simulink model "Autopilot_q_full_5may_new1"  (R2020a)
settings: Solver=ode4  StartTime=0.0  StopTime=300  FixedStep=0.01  RelTol=1e-3
undefined symbols (not defined in the file or in its folder): Aero_cofficients, Atmosphere_pert, Atmospheric_model, Counter_sensor_model, Earth, error_global, flags_global, Guidance_Flags_global, INT_global, param_guidance, Payload_data, Plane_state_mode_finish_catcher_ftr_mode, Plane_state_mode_finish_catcher_fw_mode, Plane_state_mode_finish_catcher_q_mode, Plane_state_mode_finish_catcher_rtr_mode, Plane_state_store, propulsion_model, propulsion_model_int, Structural_data, Thrust_data_store, time_global, WGS84, Wind_data, Wind_model_int, Wind_pert_factor
libraries: simulink x33, aerolibactuator x15, cstblocks x3, aerolibatmos2 x2, aerolibfltsims x1, aerolibtransform2 x1, shared6dof x1
(part 1 of 10)
settings Model: SimulationMode=accelerator  Creator=rrpat  LastModifiedBy=VTOL_HYD
settings DataIOCC: ReturnWorkspaceOutputs=off
settings DebuggingCC: ArithmeticOperatorsInVariantConditions=warning
settings SFSimCC: CustomCodeUndefinedFunction=UseInterfaceOnly

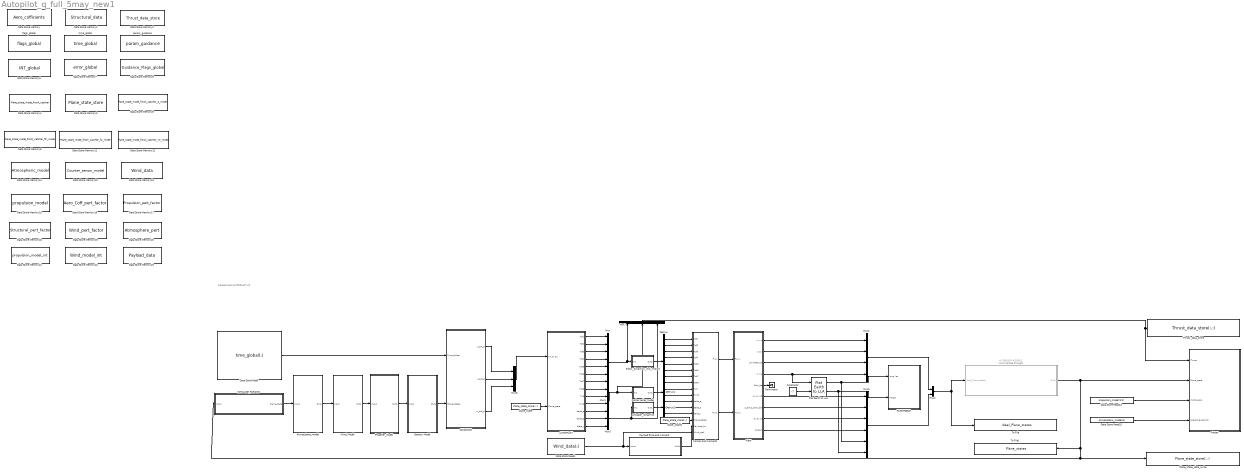
== system Autopilot_q_full_5may_new1 ==
  note: AKSHAYAAN AUTOPILOT V2
  "AUTOPILOT " : Subsystem
  Actuator_dynamics : Subsystem
  All SENSOR MODEL2 : Subsystem  Commented=through  TreatAsAtomicUnit=on
  Atmosphere_model : Subsystem
  Battery Model : Subsystem
  Constant2 : Constant  Value=-7
  Data Store Memory : DataStoreMemory  Priority=1  DataStoreName=Aero_cofficients  ReadBeforeWriteMsg=warning  WriteAfterWriteMsg=warning  WriteAfterReadMsg=warning  InitialValue=[0 0 0 0 0 0 0 0 0;0 0 0 0 0 0 0 0 0;0 0 0 0 0 0 0 0 0;0 0 0 0 0 0 0 0 0;0 0 0 0 0 0 0 0 0;0 0 0 0 0 0 0 0 0]  VectorParams1D=off  ShowAdditionalParam=off
  Data Store Memory1 : DataStoreMemory  Priority=2  DataStoreName=Structural_data  ReadBeforeWriteMsg=warning  WriteAfterWriteMsg=warning  WriteAfterReadMsg=warning  InitialValue=[25.0,0,0,0,0,0,0,0,0,0,0,0,0,0,0,0,0,0,0,0,0,0,0,0]  VectorParams1D=off  ShowAdditionalParam=off  OutDataTypeStr=double
  Data Store Memory10 : DataStoreMemory  Priority=17  DataStoreName=Counter_sensor_model  ReadBeforeWriteMsg=warning  WriteAfterWriteMsg=warning  WriteAfterReadMsg=warning  InitialValue=[0,0,0,0,1,1,1,1]  ShowAdditionalParam=off
  Data Store Memory11 : DataStoreMemory  Priority=15  DataStoreName=Plane_state_mode_finish_catcher_fw_mode  ReadBeforeWriteMsg=warning  WriteAfterWriteMsg=warning  WriteAfterReadMsg=warning  InitialValue=[0,0,0,0,0,0,0,0,0,0,0,0,0,0]  ShowAdditionalParam=off
  Data Store Memory12 : DataStoreMemory  Priority=14  DataStoreName=Plane_state_mode_finish_catcher_rtr_mode  ReadBeforeWriteMsg=warning  WriteAfterWriteMsg=warning  WriteAfterReadMsg=warning  InitialValue=[0,0,0,0,0,0,0,0,0,0,0,0,0,0]  ShowAdditionalParam=off
  Data Store Memory13 : DataStoreMemory  Priority=18  DataStoreName=Wind_data  ReadBeforeWriteMsg=warning  WriteAfterWriteMsg=warning  WriteAfterReadMsg=warning  InitialValue=[0,0,0]  ShowAdditionalParam=off
  Data Store Memory14 : DataStoreMemory  Priority=16  DataStoreName=Atmospheric_model  ReadBeforeWriteMsg=warning  WriteAfterWriteMsg=warning  WriteAfterReadMsg=warning  InitialValue=[0,0,0,0]  ShowAdditionalParam=off
  Data Store Memory15 : DataStoreMemory  Priority=19  DataStoreName=propulsion_model  ReadBeforeWriteMsg=warning  WriteAfterWriteMsg=warning  WriteAfterReadMsg=warning  InitialValue=[0,0,0,0]  ShowAdditionalParam=off
  Data Store Memory16 : DataStoreMemory  Priority=20  DataStoreName=Aero_Coff_pert_factor  ReadBeforeWriteMsg=warning  WriteAfterWriteMsg=warning  WriteAfterReadMsg=warning  InitialValue=[1 1 1 1 1 1 1 1 1;1 1 1 1 1 1 1 1 1;1 1 1 1 1 1 1 1 1;1 1 1 1 1 1 1 1 1;1 1 1 1 1 1 1 1 1;1 1 1 1 1 1 1 1 1]  VectorParams1D=off  ShowAdditionalParam=off
  Data Store Memory17 : DataStoreMemory  Priority=21  DataStoreName=Propulsion_pert_factor  ReadBeforeWriteMsg=warning  WriteAfterWriteMsg=warning  WriteAfterReadMsg=warning  InitialValue=[1,1,1,1]  ShowAdditionalParam=off
  Data Store Memory18 : DataStoreMemory  Priority=22  DataStoreName=Structural_pert_factor  ReadBeforeWriteMsg=warning  WriteAfterWriteMsg=warning  WriteAfterReadMsg=warning  InitialValue=[1,1,1,1,1,1,1,1,1,1,1,1,1,1,1,1,1,1,1,1,1,1,1,1]  VectorParams1D=off  ShowAdditionalParam=off  OutDataTypeStr=double
  Data Store Memory19 : DataStoreMemory  Priority=23  DataStoreName=Wind_pert_factor  ReadBeforeWriteMsg=warning  WriteAfterWriteMsg=warning  WriteAfterReadMsg=warning  InitialValue=[1,1,1]  ShowAdditionalParam=off
  Data Store Memory2 : DataStoreMemory  Priority=3  DataStoreName=Thrust_data_store  ReadBeforeWriteMsg=warning  WriteAfterWriteMsg=warning  WriteAfterReadMsg=warning  InitialValue=[0,0,0,0,0,0,0,0,0,0,0,0,0]  VectorParams1D=off  ShowAdditionalParam=off
  Data Store Memory20 : DataStoreMemory  Priority=24  DataStoreName=Atmosphere_pert  ReadBeforeWriteMsg=warning  WriteAfterWriteMsg=warning  WriteAfterReadMsg=warning  InitialValue=[1,1,1,1]  ShowAdditionalParam=off
  Data Store Memory21 : DataStoreMemory  Priority=27  DataStoreName=propulsion_model_int  ReadBeforeWriteMsg=warning  WriteAfterWriteMsg=warning  WriteAfterReadMsg=warning  InitialValue=[0,0,0,0]  ShowAdditionalParam=off
  Data Store Memory22 : DataStoreMemory  Priority=26  DataStoreName=Wind_model_int  ReadBeforeWriteMsg=warning  WriteAfterWriteMsg=warning  WriteAfterReadMsg=warning  InitialValue=[0,0,0,0,0,0,0,0,0,0]  ShowAdditionalParam=off
  Data Store Memory23 : DataStoreMemory  Priority=25  DataStoreName=Payload_data  ReadBeforeWriteMsg=warning  WriteAfterWriteMsg=warning  WriteAfterReadMsg=warning  InitialValue=[0,0,0,0,0,0,0,0,0,0,0,0,0,0,0,0,0,0,0,0,0,0,0,0,0,0,0,0,0,0]  ShowAdditionalParam=off
  Data Store Memory3 : DataStoreMemory  Priority=11  DataStoreName=Plane_state_store  ReadBeforeWriteMsg=warning  WriteAfterWriteMsg=warning  WriteAfterReadMsg=warning  InitialValue=[0,0,0,0,0,0,0,0,0,0,0,0,0,0,0,0,0,0,0,0,0,0,0,0,0,0,0]  VectorParams1D=off  ShowAdditionalParam=off
  Data Store Memory4 : DataStoreMemory  Priority=10  DataStoreName=Plane_state_mode_finish_catcher  ReadBeforeWriteMsg=warning  WriteAfterWriteMsg=warning  WriteAfterReadMsg=warning  InitialValue=[0,0,0,0,0,0,0,0,0,0,0,0,0,0]  ShowAdditionalParam=off
  Data Store Memory5 : DataStoreMemory  Priority=7  DataStoreName=INT_global  ReadBeforeWriteMsg=warning  WriteAfterWriteMsg=warning  WriteAfterReadMsg=warning  InitialValue=[0,0,0,0,0,0,0,0,0,0,0,0,0,0]  ShowAdditionalParam=off
  Data Store Memory6 : DataStoreMemory  Priority=9  DataStoreName=Guidance_Flags_global  ReadBeforeWriteMsg=warning  WriteAfterWriteMsg=warning  WriteAfterReadMsg=warning  InitialValue=[0,0,0,0,0,0,0,0,0,0,0,0,0,0,0,0,0,0,0,0,0,0,0,0,0,0,0,0,0,0,0,0,0,0,0,0,0,0,0,0,0,0,0,0,0,0,0,0,0,0,0]  VectorParams1D=off  ShowAdditionalParam=off
  Data Store Memory7 : DataStoreMemory  Priority=8  DataStoreName=error_global  ReadBeforeWriteMsg=warning  WriteAfterWriteMsg=warning  WriteAfterReadMsg=warning  InitialValue=[0,0,0,0,0,0]  ShowAdditionalParam=off
  Data Store Memory8 : DataStoreMemory  Priority=12  DataStoreName=Plane_state_mode_finish_catcher_q_mode  ReadBeforeWriteMsg=warning  WriteAfterWriteMsg=warning  WriteAfterReadMsg=warning  InitialValue=[0,0,0,0,0,0,0,0,0,0,0,0,0,0]  ShowAdditionalParam=off
  Data Store Memory9 : DataStoreMemory  Priority=13  DataStoreName=Plane_state_mode_finish_catcher_ftr_mode  ReadBeforeWriteMsg=warning  WriteAfterWriteMsg=warning  WriteAfterReadMsg=warning  InitialValue=[0,0,0,0,0,0,0,0,0,0,0,0,0,0]  ShowAdditionalParam=off
  Data Store Read : DataStoreRead  DataStoreName=time_global  DataStoreElements=time_global(:)
  Data Store Read1 : DataStoreRead  DataStoreName=Wind_data  SampleTime=0.01  DataStoreElements=Wind_data(:)
  Data Store Read13 : DataStoreRead  DataStoreName=propulsion_model  DataStoreElements=propulsion_model(1:2)
  Data Store Read15 : DataStoreRead  DataStoreName=Atmospheric_model  DataStoreElements=Atmospheric_model(4)
  Demux : Demux  Outputs=8
  Demux1 : Demux  Outputs=2
  Demux2 : Demux  Outputs=3
  FLIGHTGEAR : Subsystem
  Flat Earth to LLA : aerolibtransform2/Flat Earth to LLA  units=Metric (MKS)  ptype=Earth (WGS84)  F=1/298.257223563  R=6378137  refPosPort=off  LL0=[37.6188056,-122.3754167 ]  psi=0
  Forces and moments : Subsystem
  GUIDANCE : Subsystem
  INITIALISE_PARAMS : Subsystem  Priority=28
  Mux : Mux  Inputs=8
  Mux1 : Mux  Inputs=2
  Mux2 : Mux
  Mux3 : Mux  Inputs=6
  Mux4 : Mux  Inputs=2
  Mux5 : Mux  Inputs=3
  Mux6 : Mux  Inputs=3
  Mux7 : Mux  Inputs=3
  Payload force and moment : Subsystem
  Plane_state_data_write : DataStoreWrite  DataStoreName=Plane_state_store  DataStoreElements=Plane_state_store(:,:)
  Plant : Subsystem
  Plotter : Subsystem
  Propeller_Model : Subsystem
  Pusher.puller model : Subsystem
  Rotor_dynamics_vtol_motors : Subsystem
  Terminator : Terminator
  Thrust_data_store : DataStoreWrite  DataStoreName=Thrust_data_store  DataStoreElements=Thrust_data_store(:,:)
  To File : ToFile  Filename=ideal_Plane_states
  To File1 : ToFile  Filename=Plane_states  SaveFormat=Timeseries
  Wind_Model : Subsystem
  flags_global : DataStoreMemory  Priority=4  DataStoreName=flags_global  ReadBeforeWriteMsg=warning  WriteAfterWriteMsg=warning  WriteAfterReadMsg=warning  InitialValue=[0,0,0,0,0,0,0,0,0,0,0,0,0,0,0,1,1,1,1,1,1,0,0,0,1,1,0,0]  ShowAdditionalParam=off
  param_guidance : DataStoreMemory  Priority=6  DataStoreName=param_guidance  ReadBeforeWriteMsg=warning  WriteAfterWriteMsg=warning  WriteAfterReadMsg=warning  InitialValue=[0,0,0,0]  ShowAdditionalParam=off
  plane_state : DataStoreRead  DataStoreName=Plane_state_store  SampleTime=0.01  DataStoreElements=Plane_state_store(:,:)
  plane_state1 : DataStoreRead  DataStoreName=Plane_state_store  SampleTime=0.01  DataStoreElements=Plane_state_store(:,:)
  time_global : DataStoreMemory  Priority=5  DataStoreName=time_global  ReadBeforeWriteMsg=warning  WriteAfterWriteMsg=warning  WriteAfterReadMsg=warning  InitialValue=[0,0,0,0,0,0,0,0,0]  ShowAdditionalParam=off
  wires:
  "AUTOPILOT "/6(Tzb6) -> Mux/6
  Demux/3 -> Forces and moments/3("Tzf3 ")
  Plant/9(Output) -> Mux3/4
  INITIALISE_PARAMS/1(Plane_state) -> Atmosphere_model/1(Input)
  "AUTOPILOT "/5(Tzb5) -> Mux/5
  Demux2/3 -> Forces and moments/13(delta_r)
  Data Store Read15/1 -> Plotter/4(operating_density)
  Demux/7 -> Forces and moments/7(Tzb7)
  Data Store Read13/1 -> Plotter/3(motor_para)
  Pusher.puller model/1(Out1) -> Demux1/1
  Plant/8(ax,ay,az) -> Mux3/3
  Flat Earth to LLA/1 -> FLIGHTGEAR/1("long, lat"), Mux3/5
  Demux1/1 -> Forces and moments/9(Tx9)
  Demux/8 -> Forces and moments/8(Tzb8)
  Demux/4 -> Forces and moments/4(Tzf4)
  Mux7/1 -> Thrust_data_store/1, Plotter/1(Thrust)
  Demux/1 -> Forces and moments/1(Tzf1)
  Mux6/1 -> "AUTOPILOT "/1(ax,ay,az)
  Mux5/1 -> Mux7/3, Actuator_dynamics/1(In1)
  Demux1/2 -> Forces and moments/10(Tx10)
  Mux/1 -> Mux7/1, Rotor_dynamics_vtol_motors/1(In1)
  Forces and moments/1(Fxyz) -> Plant/1(Fxyz)
  Demux/5 -> Forces and moments/5(Tzb5)
  Demux/6 -> Forces and moments/6(Tzb6)
  "AUTOPILOT "/7(Tzb7) -> Mux/7
  Forces and moments/2(Mxyz) -> Plant/2(Mxyz)
  GUIDANCE/1(u_dot_d) -> Mux6/1
  "AUTOPILOT "/11(delta_e) -> Mux5/1
  GUIDANCE/3(w_dot_d) -> Mux6/3
  "AUTOPILOT "/8(Tzb8) -> Mux/8
  Mux3/1 -> Mux4/2
  Actuator_dynamics/1(Out1) -> Demux2/1
  "AUTOPILOT "/13(delta_r) -> Mux5/3
  "AUTOPILOT "/10(Tx10) -> Mux1/2
  "AUTOPILOT "/12(delta_a) -> Mux5/2
  Rotor_dynamics_vtol_motors/1(Out1) -> Demux/1
  Demux2/1 -> Forces and moments/11(delta_e)
  "AUTOPILOT "/4(Tzf4) -> Mux/4
  Mux1/1 -> Pusher.puller model/1(In1), Mux7/2
  Plant/5(Dcm_be) -> Terminator/1
  Plant/3(phi,theta,psi) -> Mux2/3
  Demux2/2 -> Forces and moments/12(delta_a)
  Plant/1(u,v,w) -> Mux2/1
  "AUTOPILOT "/2(Tzf2) -> Mux/2
  Plant/2(p,q,r) -> Mux2/2
  "AUTOPILOT "/1(Tzf1) -> Mux/1
  "AUTOPILOT "/9(Tx9) -> Mux1/1
  Flat Earth to LLA/2 -> Mux3/6, FLIGHTGEAR/2(height)
  Plant/4(X,Y,Z) -> Mux2/4, Flat Earth to LLA/1
  Plant/7(p_dot,q_dot,r_dot) -> Mux3/2
  Demux/2 -> Forces and moments/2(Tzf2)
  Data Store Read/1 -> GUIDANCE/1(Time global)
  Constant2/1 -> Flat Earth to LLA/2
  GUIDANCE/2(v_dot_d) -> Mux6/2
  Plant/6(VX,VY,VZ) -> Mux3/1
  "AUTOPILOT "/3(Tzf3) -> Mux/3
  Mux2/1 -> Mux4/1
  Mux4/1 -> All SENSOR MODEL2/1(ideal_Plane_states), To File/1
  Data Store Read1/1 -> Forces and moments/16(Wind_ned), Payload force and moment/1(Input)
  Payload force and moment/1(Out1) -> Forces and moments/15(Payload_fm)
  All SENSOR MODEL2/1(Out1) -> Plane_state_data_write/1, INITIALISE_PARAMS/1(Input), To File1/1, Plotter/2(Plane_state)
  Atmosphere_model/1(Out1) -> Wind_Model/1(Input)
  Propeller_Model/1(Out1) -> Battery Model/1(Input)
  Wind_Model/1(Out1) -> Propeller_Model/1(Input)
  Battery Model/1(Out1) -> GUIDANCE/2(Plane_states)
  plane_state/1 -> "AUTOPILOT "/2(Plane_state)
  plane_state1/1 -> Forces and moments/14(Plane_states)

== system Autopilot_q_full_5may_new1/AUTOPILOT  ==
  ax,ay,az : Inport  SampleTime=0.01
  Plane_state : Inport  Port=2  SampleTime=0.01
  Autopilot Fixed wing mode : Subsystem  TreatAsAtomicUnit=on
  Autopilot Quad mode : Subsystem  TreatAsAtomicUnit=on
  Autopilot Transition mode : Subsystem  TreatAsAtomicUnit=on
  Data Store Read : DataStoreRead  DataStoreName=flags_global  SampleTime=0.01  DataStoreElements=flags_global(3)
  Data Store Read1 : DataStoreRead  DataStoreName=flags_global  SampleTime=0.01  DataStoreElements=flags_global(4)
  Data Store Read2 : DataStoreRead  DataStoreName=flags_global  SampleTime=0.01  DataStoreElements=flags_global(5)
  Demux : Demux  Outputs=13
  Display : Display
  Display1 : Display
  Display2 : Display
  If : If  NumInputs=3  IfExpression=u1 == 1  ElseIfExpressions=u2 == 1, u3==1  ShowElse=off
  Mux : Mux  Inputs=13
  Mux1 : Mux  Inputs=13
  Mux2 : Mux  Inputs=13
  Subsystem : Subsystem
  Switch : Switch  Criteria=u2 ~= 0
  Switch1 : Switch  Criteria=u2 ~= 0
  Tzf1 : Outport  VectorParamsAs1DForOutWhenUnconnected=off
  Tzf2 : Outport  Port=2  VectorParamsAs1DForOutWhenUnconnected=off
  Tzf3 : Outport  Port=3  VectorParamsAs1DForOutWhenUnconnected=off
  Tzf4 : Outport  Port=4  VectorParamsAs1DForOutWhenUnconnected=off
  Tzb5 : Outport  Port=5  VectorParamsAs1DForOutWhenUnconnected=off
  Tzb6 : Outport  Port=6  VectorParamsAs1DForOutWhenUnconnected=off
  Tzb7 : Outport  Port=7  VectorParamsAs1DForOutWhenUnconnected=off
  Tzb8 : Outport  Port=8  VectorParamsAs1DForOutWhenUnconnected=off
  Tx9 : Outport  Port=9  VectorParamsAs1DForOutWhenUnconnected=off
  Tx10 : Outport  Port=10  VectorParamsAs1DForOutWhenUnconnected=off
  delta_e : Outport  Port=11  VectorParamsAs1DForOutWhenUnconnected=off
  delta_a : Outport  Port=12  VectorParamsAs1DForOutWhenUnconnected=off
  delta_r : Outport  Port=13  VectorParamsAs1DForOutWhenUnconnected=off
  wires:
  Plane_state/1 -> Autopilot Fixed wing mode/2(Plane_states), Autopilot Transition mode/2(Plane_state), Autopilot Quad mode/2(Plane_states)
  ax,ay,az/1 -> Autopilot Fixed wing mode/1(ax_d,ay_d,az_d), Autopilot Quad mode/1(ax_d,ay_d,az_d), Autopilot Transition mode/1(ax,ay,az)
  If/1 -> Autopilot Quad mode/Action
  If/3 -> Autopilot Fixed wing mode/Action
  Autopilot Quad mode/1(Tzf1) -> Mux/1
  Autopilot Quad mode/2(Tzf2) -> Mux/2
  Autopilot Quad mode/3(Tzf3) -> Mux/3
  Autopilot Quad mode/4(Tzf4) -> Mux/4
  Autopilot Quad mode/5(Tzb5) -> Mux/5
  Autopilot Quad mode/6(Tzb6) -> Mux/6
  Autopilot Quad mode/7(Tzb7) -> Mux/7
  Autopilot Quad mode/8(Tzb8) -> Mux/8
  Autopilot Quad mode/9(Tx9) -> Mux/9
  Autopilot Quad mode/10(Tx10) -> Mux/10
  Autopilot Quad mode/11(delta_e) -> Mux/11
  Autopilot Quad mode/12(delta_a) -> Mux/12
  Autopilot Quad mode/13(delta_r) -> Mux/13
  Autopilot Transition mode/1(Tzf1) -> Mux1/1
  Autopilot Transition mode/2(Tzf2) -> Mux1/2
  Autopilot Transition mode/3(Tzf3) -> Mux1/3
  Autopilot Transition mode/4(Tzf4) -> Mux1/4
  Autopilot Transition mode/5(Tzb5) -> Mux1/5
  Autopilot Transition mode/6(Tzb6) -> Mux1/6
  Autopilot Transition mode/7(Tzb7) -> Mux1/7
  Autopilot Transition mode/8(Tzb8) -> Mux1/8
  Autopilot Transition mode/9(Tx9) -> Mux1/9
  Autopilot Transition mode/10(Tx10) -> Mux1/10
  Autopilot Transition mode/11(delta_e) -> Mux1/11
  Autopilot Transition mode/12(delta_a) -> Mux1/12
  Autopilot Transition mode/13(delta_r) -> Mux1/13
  Mux/1 -> Switch/1
  Subsystem/1(Out1) -> Display1/1, If/1, Switch/2
  Subsystem/2(Out2) -> If/2, Display2/1
  Switch1/1 -> Switch/3
  Switch/1 -> Demux/1
  Demux/8 -> Tzb8/1
  Demux/2 -> Tzf2/1
  Demux/10 -> Tx10/1
  Demux/6 -> Tzb6/1
  Demux/5 -> Tzb5/1
  Demux/7 -> Tzb7/1
  Demux/4 -> Tzf4/1
  Demux/11 -> delta_e/1
  Demux/3 -> Tzf3/1
  Demux/9 -> Tx9/1
  Demux/1 -> Tzf1/1
  Demux/13 -> delta_r/1
  Demux/12 -> delta_a/1
  Subsystem/3(Out3) -> Display/1, Switch1/2, If/3
  If/2 -> Autopilot Transition mode/Action
  Autopilot Fixed wing mode/1(Tzf1) -> Mux2/1
  Autopilot Fixed wing mode/2(Tzf2) -> Mux2/2
  Autopilot Fixed wing mode/3(Tzf3) -> Mux2/3
  Autopilot Fixed wing mode/4(Tzf4) -> Mux2/4
  Autopilot Fixed wing mode/5(Tzb5) -> Mux2/5
  Autopilot Fixed wing mode/6(Tzb6) -> Mux2/6
  Autopilot Fixed wing mode/7(Tzb7) -> Mux2/7
  Autopilot Fixed wing mode/8(Tzb8) -> Mux2/8
  Autopilot Fixed wing mode/9(Tx9) -> Mux2/9
  Autopilot Fixed wing mode/10(Tx10) -> Mux2/10
  Autopilot Fixed wing mode/11(delta_e) -> Mux2/11
  Autopilot Fixed wing mode/12(delta_a) -> Mux2/12
  Autopilot Fixed wing mode/13(delta_r) -> Mux2/13
  Mux2/1 -> Switch1/1
  Mux1/1 -> Switch1/3
  Data Store Read/1 -> Subsystem/1(In1)
  Data Store Read1/1 -> Subsystem/2(In2)
  Data Store Read2/1 -> Subsystem/3(In3)

== system Autopilot_q_full_5may_new1/Actuator_dynamics ==
  In1 : Inport
  Actutator dynamics : aerolibactuator/Nonlinear Second-Order Actuator  wn_fin=200  z_fin=0.5  fin_max=20*pi/180  fin_min=-20*pi/180  fin_maxrate=5000*pi/180  fin_act_0=0  fin_act_vel=0
      settings: SourceProductBaseCode=AE
  Out1 : Outport  SampleTime=0.01  VectorParamsAs1DForOutWhenUnconnected=off
  wires:
  Actutator dynamics/1 -> Out1/1
  In1/1 -> Actutator dynamics/1

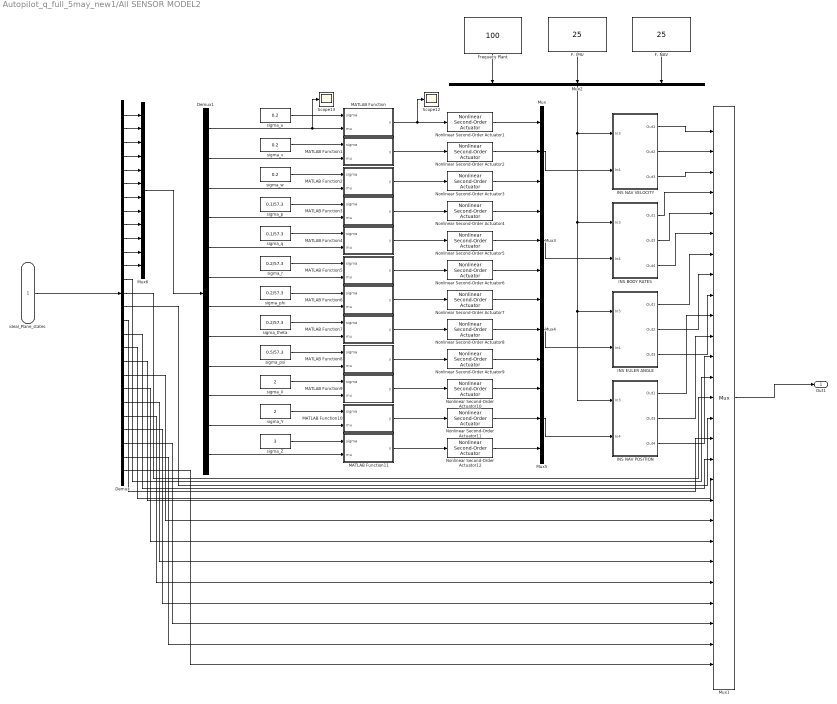
== system Autopilot_q_full_5may_new1/All SENSOR MODEL2 ==
  ideal_Plane_states : Inport
  " F. IMU" : Constant  Value=25
  " F. NAV" : Constant  Value=25
  Demux : Demux  Outputs=27
  Demux1 : Demux  Outputs=12
  Frequecy Plant : Constant  Value=100
  INS BODY RATES : Subsystem
  INS EULER ANGLE : Subsystem
  INS NAV POSITION : Subsystem
  "INS NAV VELOCITY  " : Subsystem
  MATLAB Function : MATLAB Function  TreatAsAtomicUnit=on
  MATLAB Function1 : MATLAB Function  TreatAsAtomicUnit=on
  MATLAB Function10 : MATLAB Function  TreatAsAtomicUnit=on
  MATLAB Function11 : MATLAB Function  TreatAsAtomicUnit=on
  MATLAB Function2 : MATLAB Function
  MATLAB Function3 : MATLAB Function  TreatAsAtomicUnit=on
  MATLAB Function4 : MATLAB Function  TreatAsAtomicUnit=on
  MATLAB Function5 : MATLAB Function  TreatAsAtomicUnit=on
  MATLAB Function6 : MATLAB Function  TreatAsAtomicUnit=on
  MATLAB Function7 : MATLAB Function  TreatAsAtomicUnit=on
  MATLAB Function8 : MATLAB Function  TreatAsAtomicUnit=on
  MATLAB Function9 : MATLAB Function  TreatAsAtomicUnit=on
  Mux{,2..5} (5 alike) : Mux  Inputs=3
  Mux1 : Mux  Inputs=27
  Mux6 : Mux  Inputs=12
  Nonlinear Second-Order Actuator1 : aerolibactuator/Nonlinear Second-Order Actuator  wn_fin=100  z_fin=0.5  fin_max=50000000  fin_min=-5000000  fin_maxrate=16*9.81  fin_act_0=0  fin_act_vel=0
      settings: SourceProductBaseCode=AE
  Nonlinear Second-Order Actuator10 : aerolibactuator/Nonlinear Second-Order Actuator  wn_fin=33  z_fin=0.5  fin_max=50000000  fin_min=-5000000  fin_maxrate=200  fin_act_0=0  fin_act_vel=0
      settings: SourceProductBaseCode=AE
  Nonlinear Second-Order Actuator11 : aerolibactuator/Nonlinear Second-Order Actuator  wn_fin=33  z_fin=0.5  fin_max=50000000  fin_min=-5000000  fin_maxrate=200  fin_act_0=0  fin_act_vel=0
      settings: SourceProductBaseCode=AE
  Nonlinear Second-Order Actuator12 : aerolibactuator/Nonlinear Second-Order Actuator  wn_fin=33  z_fin=0.5  fin_max=50000000  fin_min=-5000000  fin_maxrate=200  fin_act_0=0  fin_act_vel=0
      settings: SourceProductBaseCode=AE
  Nonlinear Second-Order Actuator2 : aerolibactuator/Nonlinear Second-Order Actuator  wn_fin=100  z_fin=0.5  fin_max=50000000  fin_min=-5000000  fin_maxrate=16*9.81  fin_act_0=0  fin_act_vel=0
      settings: SourceProductBaseCode=AE
  Nonlinear Second-Order Actuator3 : aerolibactuator/Nonlinear Second-Order Actuator  wn_fin=100  z_fin=0.5  fin_max=50000000  fin_min=-5000000  fin_maxrate=16*9.81  fin_act_0=0  fin_act_vel=0
      settings: SourceProductBaseCode=AE
  Nonlinear Second-Order Actuator4 : aerolibactuator/Nonlinear Second-Order Actuator  wn_fin=300  z_fin=0.5  fin_max=50000000  fin_min=-5000000  fin_maxrate=1000/57.3  fin_act_0=0  fin_act_vel=0
      settings: SourceProductBaseCode=AE
  Nonlinear Second-Order Actuator5 : aerolibactuator/Nonlinear Second-Order Actuator  wn_fin=300  z_fin=0.5  fin_max=50000000  fin_min=-5000000  fin_maxrate=1000/57.3  fin_act_0=0  fin_act_vel=0
      settings: SourceProductBaseCode=AE
  Nonlinear Second-Order Actuator6 : aerolibactuator/Nonlinear Second-Order Actuator  wn_fin=300  z_fin=0.5  fin_max=50000000  fin_min=-5000000  fin_maxrate=1000/57.3  fin_act_0=0  fin_act_vel=0
      settings: SourceProductBaseCode=AE
  Nonlinear Second-Order Actuator7 : aerolibactuator/Nonlinear Second-Order Actuator  wn_fin=100  z_fin=0.5  fin_max=50000000  fin_min=-5000000  fin_maxrate=450/57.3  fin_act_0=0  fin_act_vel=0
      settings: SourceProductBaseCode=AE
  Nonlinear Second-Order Actuator8 : aerolibactuator/Nonlinear Second-Order Actuator  wn_fin=100  z_fin=0.5  fin_max=50000000  fin_min=-5000000  fin_maxrate=450/57.3  fin_act_0=0  fin_act_vel=0
      settings: SourceProductBaseCode=AE
  Nonlinear Second-Order Actuator9 : aerolibactuator/Nonlinear Second-Order Actuator  wn_fin=100  z_fin=0.5  fin_max=50000000  fin_min=-5000000  fin_maxrate=450/57.3  fin_act_0=0  fin_act_vel=0
      settings: SourceProductBaseCode=AE
  Scope12 : Scope
  Scope13 : Scope
  sigma_X : Constant  Value=2
  sigma_Y : Constant  Value=2
  sigma_Z : Constant  Value=3
  sigma_p : Constant  Value=0.1/57.3
  sigma_phi : Constant  Value=0.2/57.3
  sigma_psi : Constant  Value=0.5/57.3
  sigma_q : Constant  Value=0.1/57.3
  sigma_r : Constant  Value=0.2/57.3
  sigma_theta : Constant  Value=0.2/57.3
  sigma_u : Constant  Value=0.2
  sigma_v : Constant  Value=0.2
  sigma_w : Constant  Value=0.2
  Out1 : Outport  VectorParamsAs1DForOutWhenUnconnected=off
  wires:
  Mux1/1 -> Out1/1
  Demux/27 -> Mux1/27
  Demux/26 -> Mux1/26
  Demux/25 -> Mux1/25
  Demux/24 -> Mux1/24
  Demux/23 -> Mux1/23
  Demux/22 -> Mux1/22
  Demux/21 -> Mux1/21
  Demux/20 -> Mux1/20
  Demux/19 -> Mux1/19
  Demux/18 -> Mux1/18
  Demux/17 -> Mux1/17
  Demux/16 -> Mux1/16
  Demux/15 -> Mux1/15
  Demux/14 -> Mux1/14
  Demux/13 -> Mux1/13
  INS NAV POSITION/3(Out4) -> Mux1/12
  INS NAV POSITION/2(Out3) -> Mux1/11
  INS NAV POSITION/1(Out1) -> Mux1/10
  INS EULER ANGLE/3(Out3) -> Mux1/9
  INS EULER ANGLE/2(Out2) -> Mux1/8
  INS EULER ANGLE/1(Out1) -> Mux1/7
  INS BODY RATES/3(Out4) -> Mux1/6
  INS BODY RATES/2(Out3) -> Mux1/5
  INS BODY RATES/1(Out1) -> Mux1/4
  "INS NAV VELOCITY  "/3(Out3) -> Mux1/3
  "INS NAV VELOCITY  "/2(Out2) -> Mux1/2
  "INS NAV VELOCITY  "/1(Out1) -> Mux1/1
  Mux6/1 -> Demux1/1
  Demux/12 -> Mux6/12
  Demux/11 -> Mux6/11
  Demux/10 -> Mux6/10
  Demux/9 -> Mux6/9
  Demux/8 -> Mux6/8
  Demux/7 -> Mux6/7
  Demux/6 -> Mux6/6
  Demux/5 -> Mux6/5
  Demux/4 -> Mux6/4
  Demux/3 -> Mux6/3
  Demux/2 -> Mux6/2
  Demux/1 -> Mux6/1
  ideal_Plane_states/1 -> Demux/1
  MATLAB Function8/1(y) -> Nonlinear Second-Order Actuator9/1
  MATLAB Function7/1(y) -> Nonlinear Second-Order Actuator8/1
  sigma_q/1 -> MATLAB Function4/1(sigma)
  MATLAB Function11/1(y) -> Nonlinear Second-Order Actuator12/1
  sigma_v/1 -> MATLAB Function1/1(sigma)
  MATLAB Function9/1(y) -> Nonlinear Second-Order Actuator10/1
  MATLAB Function6/1(y) -> Nonlinear Second-Order Actuator7/1
  sigma_w/1 -> MATLAB Function2/1(sigma)
  sigma_phi/1 -> MATLAB Function6/1(sigma)
  Demux1/1 -> MATLAB Function/2(mu), Scope13/1
  MATLAB Function2/1(y) -> Nonlinear Second-Order Actuator3/1
  MATLAB Function3/1(y) -> Nonlinear Second-Order Actuator4/1
  sigma_Y/1 -> MATLAB Function10/1(sigma)
  Demux1/8 -> MATLAB Function7/2(mu)
  sigma_r/1 -> MATLAB Function5/1(sigma)
  sigma_u/1 -> MATLAB Function/1(sigma)
  Demux1/3 -> MATLAB Function2/2(mu)
  sigma_X/1 -> MATLAB Function9/1(sigma)
  MATLAB Function/1(y) -> Nonlinear Second-Order Actuator1/1, Scope12/1
  Demux1/7 -> MATLAB Function6/2(mu)
  MATLAB Function10/1(y) -> Nonlinear Second-Order Actuator11/1
  Demux1/4 -> MATLAB Function3/2(mu)
  sigma_theta/1 -> MATLAB Function7/1(sigma)
  sigma_p/1 -> MATLAB Function3/1(sigma)
  MATLAB Function5/1(y) -> Nonlinear Second-Order Actuator6/1
  Demux1/10 -> MATLAB Function9/2(mu)
  Demux1/11 -> MATLAB Function10/2(mu)
  MATLAB Function1/1(y) -> Nonlinear Second-Order Actuator2/1
  Demux1/2 -> MATLAB Function1/2(mu)
  MATLAB Function4/1(y) -> Nonlinear Second-Order Actuator5/1
  sigma_Z/1 -> MATLAB Function11/1(sigma)
  sigma_psi/1 -> MATLAB Function8/1(sigma)
  Demux1/5 -> MATLAB Function4/2(mu)
  Demux1/12 -> MATLAB Function11/2(mu)
  Demux1/9 -> MATLAB Function8/2(mu)
  Demux1/6 -> MATLAB Function5/2(mu)
  Nonlinear Second-Order Actuator1/1 -> Mux/1
  Nonlinear Second-Order Actuator2/1 -> Mux/2
  Nonlinear Second-Order Actuator3/1 -> Mux/3
  " F. IMU"/1 -> Mux2/2
  " F. NAV"/1 -> Mux2/3
  Frequecy Plant/1 -> Mux2/1
  Nonlinear Second-Order Actuator4/1 -> Mux3/1
  Nonlinear Second-Order Actuator5/1 -> Mux3/2
  Nonlinear Second-Order Actuator6/1 -> Mux3/3
  Nonlinear Second-Order Actuator7/1 -> Mux4/1
  Nonlinear Second-Order Actuator8/1 -> Mux4/2
  Nonlinear Second-Order Actuator9/1 -> Mux4/3
  Nonlinear Second-Order Actuator10/1 -> Mux5/1
  Nonlinear Second-Order Actuator11/1 -> Mux5/2
  Nonlinear Second-Order Actuator12/1 -> Mux5/3
  Mux2/1 -> "INS NAV VELOCITY  "/1(In3), INS BODY RATES/1(In3), INS NAV POSITION/1(In3), INS EULER ANGLE/1(In3)
  Mux3/1 -> INS BODY RATES/2(In4)
  Mux5/1 -> INS NAV POSITION/2(In4)
  Mux4/1 -> INS EULER ANGLE/2(In4)
  Mux/1 -> "INS NAV VELOCITY  "/2(In4)

== system Autopilot_q_full_5may_new1/Atmosphere_model ==
  Input : Inport  SampleTime=0.01
  Abs : Abs
  Data Store Read : DataStoreRead  DataStoreName=Plane_state_store  SampleTime=0.01  DataStoreElements=Plane_state_store(1,12)
  Data Store Write : DataStoreWrite  DataStoreName=Atmospheric_model  DataStoreElements=Atmospheric_model(:)
  ISA Atmosphere Model : aerolibatmos2/ISA Atmosphere Model  custom=off  g=9.80665  gamma=1.4  R=287.0531  L=0.0065  h_trop=11000  h_strat=20000  rho0=1.225  P0=101325  T0=288.15  h0=0
  Mux : Mux
  Scope{1..2,4..5} (4 alike) : Scope
  Out1 : Outport  VectorParamsAs1DForOutWhenUnconnected=off
  wires:
  Input/1 -> Out1/1
  ISA Atmosphere Model/2 -> Mux/2, Scope4/1
  Data Store Read/1 -> Abs/1
  ISA Atmosphere Model/1 -> Scope1/1, Mux/1
  Abs/1 -> ISA Atmosphere Model/1
  ISA Atmosphere Model/3 -> Mux/3, Scope5/1
  Mux/1 -> Data Store Write/1
  ISA Atmosphere Model/4 -> Scope2/1, Mux/4

== system Autopilot_q_full_5may_new1/Battery Model ==
  Input : Inport  SampleTime=0.01
  Subsystem : Subsystem
  Out1 : Outport  VectorParamsAs1DForOutWhenUnconnected=off
  wires:
  Input/1 -> Subsystem/1(In1)
  Subsystem/1(Out1) -> Out1/1

== system Autopilot_q_full_5may_new1/FLIGHTGEAR ==
  "long, lat" : Inport
  height : Inport  Port=2
  Demux : Demux  Outputs=2
  Demux1 : Demux  Outputs=3
  FlightGear Preconfigured 6DoF Animation : aerolibfltsims/FlightGear Preconfigured 6DoF Animation  xFlightGearVersion=v2017.3  DestinationIpAddress=127.0.0.1  DestinationPort=5502  SampleTime=0.01
  Flip : DSPFlip
  Mux : Mux  Inputs=6
  phi,theta,psi : DataStoreRead  DataStoreName=Plane_state_store  DataStoreElements=Plane_state_store(1,7:9)
  wires:
  Mux/1 -> FlightGear Preconfigured 6DoF Animation/1
  height/1 -> Mux/3
  "long, lat"/1 -> Flip/1
  Flip/1 -> Demux/1
  Demux/1 -> Mux/1
  Demux/2 -> Mux/2
  Demux1/1 -> Mux/4
  Demux1/2 -> Mux/5
  Demux1/3 -> Mux/6
  phi,theta,psi/1 -> Demux1/1

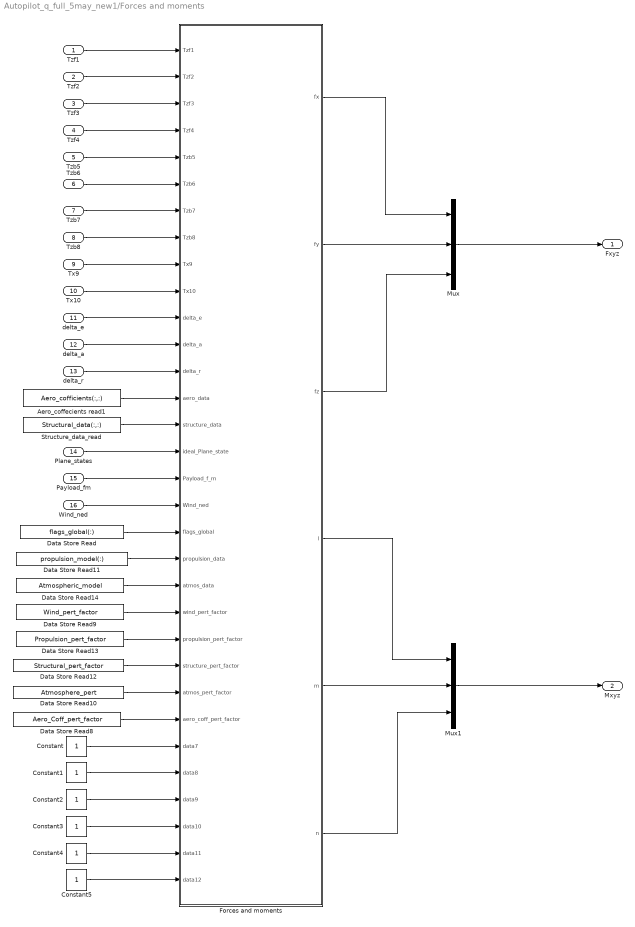
== system Autopilot_q_full_5may_new1/Forces and moments ==
  Tzf1 : Inport
  Tzf2 : Inport  Port=2
  "Tzf3 " : Inport  Port=3
  Tzf4 : Inport  Port=4
  Tzb5 : Inport  Port=5
  Tzb6 : Inport  Port=6
  Tzb7 : Inport  Port=7
  Tzb8 : Inport  Port=8
  Tx9 : Inport  Port=9
  Tx10 : Inport  Port=10
  delta_e : Inport  Port=11
  delta_a : Inport  Port=12
  delta_r : Inport  Port=13
  Plane_states : Inport  Port=14
  Payload_fm : Inport  Port=15
  Wind_ned : Inport  Port=16
  Aero_coffecients read1 : DataStoreRead  DataStoreName=Aero_cofficients  DataStoreElements=Aero_cofficients(:,:)
  Constant{,1..5} (6 alike) : Constant
  Data Store Read : DataStoreRead  DataStoreName=flags_global  DataStoreElements=flags_global(:)
  Data Store Read10 : DataStoreRead  DataStoreName=Atmosphere_pert
  Data Store Read11 : DataStoreRead  DataStoreName=propulsion_model  DataStoreElements=propulsion_model(:)
  Data Store Read12 : DataStoreRead  DataStoreName=Structural_pert_factor
  Data Store Read13 : DataStoreRead  DataStoreName=Propulsion_pert_factor
  Data Store Read14 : DataStoreRead  DataStoreName=Atmospheric_model
  Data Store Read8 : DataStoreRead  DataStoreName=Aero_Coff_pert_factor
  Data Store Read9 : DataStoreRead  DataStoreName=Wind_pert_factor
  Forces and moments : MATLAB Function  TreatAsAtomicUnit=on
  Mux : Mux  Inputs=3
  Mux1 : Mux  Inputs=3
  Structure_data_read : DataStoreRead  DataStoreName=Structural_data  DataStoreElements=Structural_data(:,:)
  Fxyz : Outport  SampleTime=0.01  VectorParamsAs1DForOutWhenUnconnected=off
  Mxyz : Outport  Port=2  SampleTime=0.01  VectorParamsAs1DForOutWhenUnconnected=off
  wires:
  Tzf2/1 -> Forces and moments/2(Tzf2)
  Tzf1/1 -> Forces and moments/1(Tzf1)
  "Tzf3 "/1 -> Forces and moments/3(Tzf3)
  Tzf4/1 -> Forces and moments/4(Tzf4)
  Tzb5/1 -> Forces and moments/5(Tzb5)
  Tzb6/1 -> Forces and moments/6(Tzb6)
  Tzb7/1 -> Forces and moments/7(Tzb7)
  Tzb8/1 -> Forces and moments/8(Tzb8)
  Tx9/1 -> Forces and moments/9(Tx9)
  Tx10/1 -> Forces and moments/10(Tx10)
  delta_e/1 -> Forces and moments/11(delta_e)
  delta_a/1 -> Forces and moments/12(delta_a)
  delta_r/1 -> Forces and moments/13(delta_r)
  Forces and moments/1(fx) -> Mux/1
  Mux1/1 -> Mxyz/1
  Mux/1 -> Fxyz/1
  Forces and moments/2(fy) -> Mux/2
  Forces and moments/3(fz) -> Mux/3
  Forces and moments/4(l) -> Mux1/1
  Forces and moments/6(n) -> Mux1/3
  Forces and moments/5(m) -> Mux1/2
  Structure_data_read/1 -> Forces and moments/15(structure_data)
  Aero_coffecients read1/1 -> Forces and moments/14(aero_data)
  Plane_states/1 -> Forces and moments/16(ideal_Plane_state)
  Payload_fm/1 -> Forces and moments/17(Payload_f_m)
  Wind_ned/1 -> Forces and moments/18(Wind_ned)
  Data Store Read/1 -> Forces and moments/19(flags_global)
  Data Store Read11/1 -> Forces and moments/20(propulsion_data)
  Data Store Read14/1 -> Forces and moments/21(atmos_data)
  Data Store Read9/1 -> Forces and moments/22(wind_pert_factor)
  Data Store Read13/1 -> Forces and moments/23(propulsion_pert_factor)
  Data Store Read12/1 -> Forces and moments/24(structure_pert_factor)
  Data Store Read10/1 -> Forces and moments/25(atmos_pert_factor)
  Data Store Read8/1 -> Forces and moments/26(aero_coff_pert_factor)
  Constant/1 -> Forces and moments/27(data7)
  Constant1/1 -> Forces and moments/28(data8)
  Constant2/1 -> Forces and moments/29(data9)
  Constant3/1 -> Forces and moments/30(data10)
  Constant4/1 -> Forces and moments/31(data11)
  Constant5/1 -> Forces and moments/32(data12)

== system Autopilot_q_full_5may_new1/GUIDANCE ==
  Time global : Inport  SampleTime=0.01
  Plane_states : Inport  Port=2  SampleTime=0.01
  "    MODE SWITCHER   &   PATH PLANNER  " : MATLAB Function  TreatAsAtomicUnit=on
  Constant{,1..5} (6 alike) : Constant
  Data Store Read : DataStoreRead  DataStoreName=flags_global  SampleTime=0.01  DataStoreElements=flags_global(:)
  Data Store Read1 : DataStoreRead  DataStoreName=param_guidance  DataStoreElements=param_guidance(:)
  Data Store Read10 : DataStoreRead  DataStoreName=Atmosphere_pert
  Data Store Read11 : DataStoreRead  DataStoreName=propulsion_model  DataStoreElements=propulsion_model(:)
  Data Store Read14 : DataStoreRead  DataStoreName=Atmospheric_model
  Data Store Read2 : DataStoreRead  DataStoreName=Guidance_Flags_global  DataStoreElements=Guidance_Flags_global(:,:)
  Data Store Read3 : DataStoreRead  DataStoreName=INT_global  DataStoreElements=INT_global(:)
  Data Store Read4 : DataStoreRead  DataStoreName=error_global  DataStoreElements=error_global(:)
  Data Store Read5 : DataStoreRead  DataStoreName=Wind_data  DataStoreElements=Wind_data(:)
  Data Store Read6 : DataStoreRead  DataStoreName=Aero_Coff_pert_factor
  Data Store Read7 : DataStoreRead  DataStoreName=Wind_pert_factor
  Data Store Read8 : DataStoreRead  DataStoreName=Propulsion_pert_factor
  Data Store Read9 : DataStoreRead  DataStoreName=Structural_pert_factor
  Data Store Write : DataStoreWrite  DataStoreName=flags_global  DataStoreElements=flags_global(:)
  Data Store Write1 : DataStoreWrite  DataStoreName=param_guidance  DataStoreElements=param_guidance(:)
  Data Store Write2 : DataStoreWrite  DataStoreName=Guidance_Flags_global  DataStoreElements=Guidance_Flags_global(:,:)
  Data Store Write3 : DataStoreWrite  DataStoreName=INT_global  DataStoreElements=INT_global(:)
  Data Store Write4 : DataStoreWrite  DataStoreName=error_global  DataStoreElements=error_global(:)
  Digital Clock : DigitalClock  SampleTime=0.01
  Mux : Mux  Inputs=2
  plane_state : DataStoreRead  DataStoreName=Plane_state_store  SampleTime=0.01  DataStoreElements=Plane_state_store(:,:)
  u_dot_d : Outport  SampleTime=0.01  VectorParamsAs1DForOutWhenUnconnected=off
  v_dot_d : Outport  Port=2  SampleTime=0.01  VectorParamsAs1DForOutWhenUnconnected=off
  w_dot_d : Outport  Port=3  SampleTime=0.01  VectorParamsAs1DForOutWhenUnconnected=off
  wires:
  plane_state/1 -> Mux/1
  Plane_states/1 -> Mux/2
  Time global/1 -> "    MODE SWITCHER   &   PATH PLANNER  "/1(Time_global)
  "    MODE SWITCHER   &   PATH PLANNER  "/1(u_dot_d) -> u_dot_d/1
  "    MODE SWITCHER   &   PATH PLANNER  "/3(w_dot_d) -> w_dot_d/1
  "    MODE SWITCHER   &   PATH PLANNER  "/4(flags_global) -> Data Store Write/1
  "    MODE SWITCHER   &   PATH PLANNER  "/2(v_dot_d) -> v_dot_d/1
  Data Store Read1/1 -> "    MODE SWITCHER   &   PATH PLANNER  "/5("param_guidance ")
  Data Store Read2/1 -> "    MODE SWITCHER   &   PATH PLANNER  "/6("guidance_global ")
  Data Store Read3/1 -> "    MODE SWITCHER   &   PATH PLANNER  "/7("INT_global ")
  Data Store Read4/1 -> "    MODE SWITCHER   &   PATH PLANNER  "/8("error_global ")
  "    MODE SWITCHER   &   PATH PLANNER  "/5(param_guidance) -> Data Store Write1/1
  "    MODE SWITCHER   &   PATH PLANNER  "/6(guidance_global) -> Data Store Write2/1
  "    MODE SWITCHER   &   PATH PLANNER  "/7(INT_global) -> Data Store Write3/1
  "    MODE SWITCHER   &   PATH PLANNER  "/8(error_global) -> Data Store Write4/1
  Mux/1 -> "    MODE SWITCHER   &   PATH PLANNER  "/4(Plane_state)
  Data Store Read/1 -> "    MODE SWITCHER   &   PATH PLANNER  "/2("flags_global ")
  Digital Clock/1 -> "    MODE SWITCHER   &   PATH PLANNER  "/3(t)
  Data Store Read5/1 -> "    MODE SWITCHER   &   PATH PLANNER  "/9(Wind_ned)
  Data Store Read11/1 -> "    MODE SWITCHER   &   PATH PLANNER  "/10(propulsion_data)
  Data Store Read14/1 -> "    MODE SWITCHER   &   PATH PLANNER  "/11(atmos_data)
  Data Store Read7/1 -> "    MODE SWITCHER   &   PATH PLANNER  "/12(wind_pert_factor)
  Data Store Read8/1 -> "    MODE SWITCHER   &   PATH PLANNER  "/13(propulsion_pert_factor)
  Data Store Read9/1 -> "    MODE SWITCHER   &   PATH PLANNER  "/14(structure_pert_factor)
  Data Store Read10/1 -> "    MODE SWITCHER   &   PATH PLANNER  "/15(atmos_pert_factor)
  Data Store Read6/1 -> "    MODE SWITCHER   &   PATH PLANNER  "/16(aero_coff_pert_factor)
  Constant/1 -> "    MODE SWITCHER   &   PATH PLANNER  "/17(data7)
  Constant1/1 -> "    MODE SWITCHER   &   PATH PLANNER  "/18(data8)
  Constant2/1 -> "    MODE SWITCHER   &   PATH PLANNER  "/19(data9)
  Constant3/1 -> "    MODE SWITCHER   &   PATH PLANNER  "/20(data10)
  Constant4/1 -> "    MODE SWITCHER   &   PATH PLANNER  "/21(data11)
  Constant5/1 -> "    MODE SWITCHER   &   PATH PLANNER  "/22(data12)

== system Autopilot_q_full_5may_new1/INITIALISE_PARAMS ==
  note: INITIALISER
  Input : Inport
  Clock : Clock
      settings: Decimation=10000
  INITIALISE MODELS : Subsystem  TreatAsAtomicUnit=on
  If : If  IfExpression=(u1) <= 0.1
  If Action Subsystem : Subsystem  TreatAsAtomicUnit=on
  Switch : Switch  Threshold=0.1
  Plane_state : Outport  VectorParamsAs1DForOutWhenUnconnected=off
  wires:
  Input/1 -> If Action Subsystem/1(In1), INITIALISE MODELS/1(In1)
  Clock/1 -> Switch/2, If/1
  Switch/1 -> Plane_state/1
  INITIALISE MODELS/1(Out1) -> Switch/1
  If Action Subsystem/1(Out1) -> Switch/3
  If/2 -> INITIALISE MODELS/Action
  If/1 -> If Action Subsystem/Action

== system Autopilot_q_full_5may_new1/Payload force and moment ==
  Input : Inport  SampleTime=0.01
  Changing Mass : Subsystem
  Data Store Read : DataStoreRead  DataStoreName=Plane_state_store  SampleTime=0.01  DataStoreElements=Plane_state_store(:,:)
  Data Store Read1 : DataStoreRead  DataStoreName=Payload_data  SampleTime=0.01  DataStoreElements=Payload_data(:)
  Data Store Read11 : DataStoreRead  DataStoreName=propulsion_model  SampleTime=0.01  DataStoreElements=propulsion_model(:)
  Data Store Read14 : DataStoreRead  DataStoreName=Atmospheric_model  SampleTime=0.01
  Data Store Write : DataStoreWrite  DataStoreName=Structural_data  DataStoreElements=Structural_data(1,1)
  Demux : Demux  Outputs=6
  MATLAB Function : MATLAB Function  TreatAsAtomicUnit=on
  Scope{,1..6} (7 alike) : Scope
  Out1 : Outport  SampleTime=0.01  VectorParamsAs1DForOutWhenUnconnected=off
  wires:
  MATLAB Function/1(Wind_f_m) -> Scope/1, Out1/1, Demux/1
  Data Store Read/1 -> Changing Mass/1(In1), MATLAB Function/1(ideal_Plane_state)
  Input/1 -> MATLAB Function/2(Wind_ned)
  Changing Mass/1(Out1) -> Data Store Write/1
  Demux/1 -> Scope1/1
  Demux/2 -> Scope2/1
  Demux/3 -> Scope3/1
  Demux/4 -> Scope4/1
  Demux/6 -> Scope5/1
  Demux/5 -> Scope6/1
  Data Store Read11/1 -> MATLAB Function/3(propulsion_data)
  Data Store Read14/1 -> MATLAB Function/4(atmos_data)
  Data Store Read1/1 -> MATLAB Function/5(payload_data)

== system Autopilot_q_full_5may_new1/Plant ==
  Fxyz : Inport  SampleTime=0.01
  Mxyz : Inport  Port=2  SampleTime=0.01
  6DOF (Euler Angles) : shared6dof/6DOF (Euler Angles)  units=Metric (MKS)  mtype=Fixed  rep=Euler Angles  xme_0=[0 0 0]  Vm_0=[0 0 0]  eul_0=[0 0 0]  pm_0=[0 0 0]  mass_0=5  mass_e=0.5  mass_f=2.0  inertia="[0.6275, 0.0, 0; 0.0, 0.564, 0; 0,  0, 1.176]"  inertia_e=eye(3)  inertia_f=2*eye(3)  k_quat=1.0  vre_flag=on  abi_flag=on  aMode=aMode  xme_statename=''  Vm_statename=''  eul_statename=''  quat_statename=''  pm_statename=''  mass_statename=''
      settings: SourceProductBaseCode=AE,PW,MT,VE,VP
  Clock : Clock
  Constant{,1..5} (6 alike) : Constant  Value=0
  Demux : Demux  Outputs=2
  Mux : Mux  Inputs=2
  Mux1 : Mux  Inputs=3
  Mux2 : Mux  Inputs=3
  Mux3 : Mux  Inputs=2
  Switch : Switch  Criteria=u2 > Threshold  Threshold=0.01
  u,v,w : Outport  VectorParamsAs1DForOutWhenUnconnected=off
  p,q,r : Outport  Port=2  VectorParamsAs1DForOutWhenUnconnected=off
  phi,theta,psi : Outport  Port=3  VectorParamsAs1DForOutWhenUnconnected=off
  X,Y,Z : Outport  Port=4  VectorParamsAs1DForOutWhenUnconnected=off
  Dcm_be : Outport  Port=5  VectorParamsAs1DForOutWhenUnconnected=off
  VX,VY,VZ : Outport  Port=6  VectorParamsAs1DForOutWhenUnconnected=off
  p_dot,q_dot,r_dot : Outport  Port=7  VectorParamsAs1DForOutWhenUnconnected=off
  ax,ay,az : Outport  Port=8  VectorParamsAs1DForOutWhenUnconnected=off
  Output : Outport  Port=9  VectorParamsAs1DForOutWhenUnconnected=off
  wires:
  6DOF (Euler Angles)/1 -> VX,VY,VZ/1
  6DOF (Euler Angles)/2 -> X,Y,Z/1
  6DOF (Euler Angles)/3 -> phi,theta,psi/1
  6DOF (Euler Angles)/4 -> Dcm_be/1
  6DOF (Euler Angles)/5 -> u,v,w/1
  6DOF (Euler Angles)/6 -> p,q,r/1
  6DOF (Euler Angles)/7 -> p_dot,q_dot,r_dot/1
  6DOF (Euler Angles)/8 -> ax,ay,az/1
  6DOF (Euler Angles)/9 -> Output/1
  Clock/1 -> Switch/2
  Fxyz/1 -> Mux/1
  Mxyz/1 -> Mux/2
  Mux/1 -> Switch/1
  Switch/1 -> Demux/1
  Demux/1 -> 6DOF (Euler Angles)/1
  Demux/2 -> 6DOF (Euler Angles)/2
  Constant/1 -> Mux1/1
  Constant1/1 -> Mux1/2
  Constant2/1 -> Mux1/3
  Constant5/1 -> Mux2/3
  Constant4/1 -> Mux2/2
  Constant3/1 -> Mux2/1
  Mux1/1 -> Mux3/1
  Mux2/1 -> Mux3/2
  Mux3/1 -> Switch/3

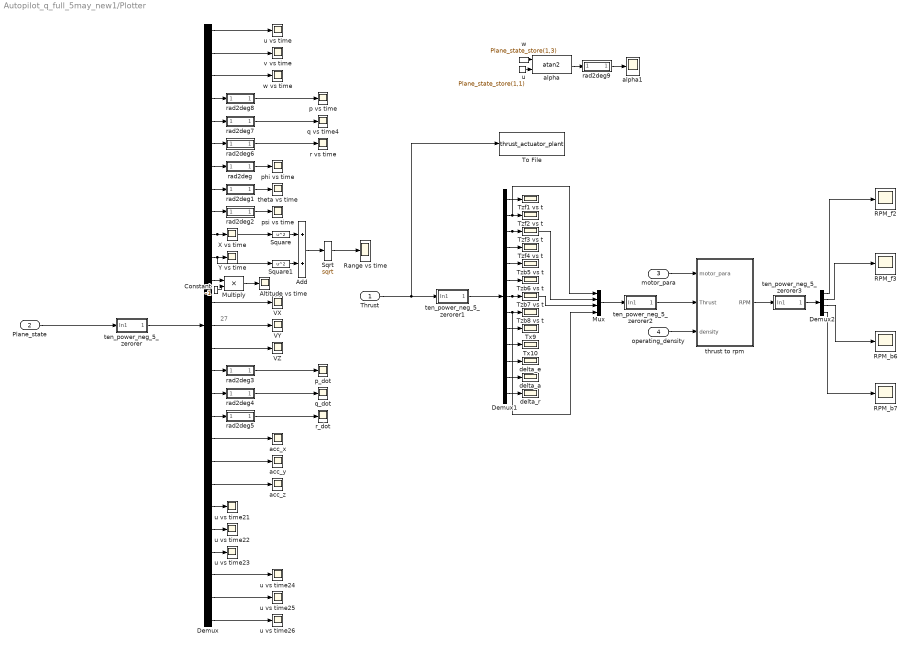
== system Autopilot_q_full_5may_new1/Plotter ==
  note: 27
  Thrust : Inport
  Plane_state : Inport  Port=2
  motor_para : Inport  Port=3
  operating_density : Inport  Port=4
  Add : Sum
  Altitude vs time : Scope
  Constant : Constant  Value=-1
  Demux : Demux  Outputs=27
  Demux1 : Demux  Outputs=13
  Demux2 : Demux
  Multiply : Product
  Mux : Mux
  RPM_b6 : Scope
  RPM_b7 : Scope
  RPM_f2 : Scope
  RPM_f3 : Scope
  Range vs time : Scope
  Sqrt : Sqrt  SaturateOnIntegerOverflow=on
  Square : Math  Operator=square  SignedPower=on  SaturateOnIntegerOverflow=on
  Square1 : Math  Operator=square  SignedPower=on  SaturateOnIntegerOverflow=on
  To File : ToFile  Filename=thrust_actuator_plant  SaveFormat=Timeseries
  Tx10 : Scope
  Tx9 : Scope
  Tzb5 vs t : Scope
  Tzb6 vs t : Scope
  Tzb7 vs t : Scope
  Tzb8 vs t : Scope
  Tzf1 vs t : Scope
  Tzf2 vs t : Scope
  Tzf3 vs t : Scope
  Tzf4 vs t : Scope
  VX : Scope
  VY : Scope
  VZ : Scope
  X vs time : Scope
  Y vs time : Scope
  acc_x : Scope
  acc_y : Scope
  acc_z : Scope
  alpha : Trigonometry  Operator=atan2
  alpha1 : Scope
  delta_a : Scope
  delta_e : Scope
  delta_r : Scope
  p vs time : Scope
  p_dot : Scope
  phi vs time : Scope
  psi vs time : Scope
  q vs time4 : Scope
  q_dot : Scope
  r vs time : Scope
  r_dot : Scope
  rad2deg : Subsystem
  rad2deg1 : Subsystem
  rad2deg2 : Subsystem
  rad2deg3 : Subsystem
  rad2deg4 : Subsystem
  rad2deg5 : Subsystem
  rad2deg6 : Subsystem
  rad2deg7 : Subsystem
  rad2deg8 : Subsystem
  rad2deg9 : Subsystem
  ten_power_neg_5_zerorer : Subsystem
  ten_power_neg_5_zerorer1 : Subsystem
  ten_power_neg_5_zerorer2 : Subsystem
  ten_power_neg_5_zerorer3 : Subsystem
  theta vs time : Scope
  thrust to rpm : Subsystem
  u : DataStoreRead  DataStoreName=Plane_state_store  DataStoreElements=Plane_state_store(1,1)
  u vs time{,21..26} (7 alike) : Scope
  v vs time : Scope
  w : DataStoreRead  DataStoreName=Plane_state_store  DataStoreElements=Plane_state_store(1,3)
  w vs time : Scope
  wires:
  Plane_state/1 -> ten_power_neg_5_zerorer/1(In1)
  Demux/1 -> u vs time/1
  Demux/2 -> v vs time/1
  Demux/3 -> w vs time/1
  Demux/4 -> rad2deg8/1(In1)
  Demux/5 -> rad2deg7/1(In1)
  Demux/6 -> rad2deg6/1(In1)
  Demux/7 -> rad2deg/1(In1)
  Demux/8 -> rad2deg1/1(In1)
  Demux/9 -> rad2deg2/1(In1)
  Demux/10 -> Square/1, X vs time/1
  Demux/11 -> Square1/1, Y vs time/1
  Demux/13 -> VX/1
  Demux/14 -> VY/1
  Demux/15 -> VZ/1
  Demux/16 -> rad2deg3/1(In1)
  Demux/17 -> rad2deg4/1(In1)
  Demux/18 -> rad2deg5/1(In1)
  Demux/19 -> acc_x/1
  Demux/20 -> acc_y/1
  Demux/21 -> acc_z/1
  Demux/22 -> u vs time21/1
  Demux/23 -> u vs time22/1
  Demux/24 -> u vs time23/1
  Demux/25 -> u vs time24/1
  Demux/26 -> u vs time25/1
  Demux/27 -> u vs time26/1
  Demux1/1 -> Tzf1 vs t/1
  Demux1/2 -> Mux/1, Tzf2 vs t/1
  Demux1/3 -> Mux/2, Tzf3 vs t/1
  Demux1/4 -> Tzf4 vs t/1
  Demux1/5 -> Tzb5 vs t/1
  Demux1/6 -> Tzb6 vs t/1
  Demux1/7 -> Mux/3, Tzb7 vs t/1
  Demux1/8 -> Mux/4, Tzb8 vs t/1
  Demux1/9 -> Tx9/1
  Demux1/10 -> Tx10/1
  Demux1/11 -> delta_e/1
  Demux1/12 -> delta_a/1
  Demux1/13 -> delta_r/1
  rad2deg/1(Out1) -> phi vs time/1
  rad2deg1/1(Out1) -> theta vs time/1
  rad2deg2/1(Out1) -> psi vs time/1
  rad2deg3/1(Out1) -> p_dot/1
  rad2deg4/1(Out1) -> q_dot/1
  rad2deg5/1(Out1) -> r_dot/1
  rad2deg6/1(Out1) -> r vs time/1
  rad2deg7/1(Out1) -> q vs time4/1
  rad2deg8/1(Out1) -> p vs time/1
  operating_density/1 -> thrust to rpm/3(density)
  motor_para/1 -> thrust to rpm/1(motor_para)
  Mux/1 -> ten_power_neg_5_zerorer2/1(In1)
  thrust to rpm/1(RPM) -> ten_power_neg_5_zerorer3/1(In1)
  Demux2/1 -> RPM_f2/1
  Demux2/3 -> RPM_b6/1
  Demux2/4 -> RPM_b7/1
  ten_power_neg_5_zerorer/1(Out1) -> Demux/1
  Thrust/1 -> To File/1, ten_power_neg_5_zerorer1/1(In1)
  ten_power_neg_5_zerorer1/1(Out1) -> Demux1/1
  ten_power_neg_5_zerorer2/1(Out1) -> thrust to rpm/2(Thrust)
  Demux2/2 -> RPM_f3/1
  ten_power_neg_5_zerorer3/1(Out1) -> Demux2/1
  Add/1 -> Sqrt/1
  Sqrt/1 -> Range vs time/1
  Square1/1 -> Add/2
  Square/1 -> Add/1
  Demux/12 -> Multiply/1
  Multiply/1 -> Altitude vs time/1
  Constant/1 -> Multiply/2
  u/1 -> alpha/2
  w/1 -> alpha/1
  alpha/1 -> rad2deg9/1(In1)
  rad2deg9/1(Out1) -> alpha1/1

== system Autopilot_q_full_5may_new1/Propeller_Model ==
  Input : Inport  SampleTime=0.01
  Data Store Read : DataStoreRead  DataStoreName=propulsion_model_int  SampleTime=0.01  DataStoreElements=propulsion_model_int(:)
  Data Store Write : DataStoreWrite  DataStoreName=propulsion_model  DataStoreElements=propulsion_model(:)
  Demux : Demux
  Divide : Product  Inputs=*/
  Multiply{,1..3} (4 alike) : Product
  Mux : Mux
  rho : DataStoreRead  DataStoreName=Atmospheric_model  SampleTime=0.01  DataStoreElements=Atmospheric_model(4)
  rho_o : Constant  Value=1.225  SampleTime=0.01
  Out1 : Outport  VectorParamsAs1DForOutWhenUnconnected=off
  wires:
  Input/1 -> Out1/1
  Data Store Read/1 -> Demux/1
  Demux/4 -> Multiply3/2
  Multiply1/1 -> Mux/2
  Demux/2 -> Multiply1/2
  Multiply2/1 -> Mux/3
  Mux/1 -> Data Store Write/1
  Divide/1 -> Multiply3/1, Multiply2/1, Multiply1/1, Multiply/1
  Demux/1 -> Multiply/2
  Multiply/1 -> Mux/1
  Multiply3/1 -> Mux/4
  rho_o/1 -> Divide/2
  rho/1 -> Divide/1
  Demux/3 -> Multiply2/2

== system Autopilot_q_full_5may_new1/Pusher.puller model ==
  In1 : Inport
  Actutator dynamics : aerolibactuator/Nonlinear Second-Order Actuator  wn_fin=200  z_fin=0.5  fin_max=50000000  fin_min=-5000000  fin_maxrate=500000000  fin_act_0=0  fin_act_vel=0
      settings: SourceProductBaseCode=AE
  Out1 : Outport  SampleTime=0.01  VectorParamsAs1DForOutWhenUnconnected=off
  wires:
  In1/1 -> Actutator dynamics/1
  Actutator dynamics/1 -> Out1/1

== system Autopilot_q_full_5may_new1/Rotor_dynamics_vtol_motors ==
  In1 : Inport
  Rotor_dynamics_vtol_motors : aerolibactuator/Nonlinear Second-Order Actuator  wn_fin=200  z_fin=0.5  fin_max=5000000  fin_min=-500000  fin_maxrate=1000000  fin_act_0=0  fin_act_vel=0
      settings: SourceProductBaseCode=AE
  Out1 : Outport  SampleTime=0.01  VectorParamsAs1DForOutWhenUnconnected=off
  wires:
  In1/1 -> Rotor_dynamics_vtol_motors/1
  Rotor_dynamics_vtol_motors/1 -> Out1/1
